simulink model "OpenLoopController"  (R2025b)
settings: configuration reference "VehicleFixed1ms" (kept outside this file)
settings Model: DataDictionary=VirtualMotoTemplate.sldd  ModifiedByFormat=The MathWorks, Inc.  Creator=The MathWorks, Inc.  LastModifiedBy=The MathWorks, Inc.
settings ConfigSetRef: SourceName=VehicleFixed1ms

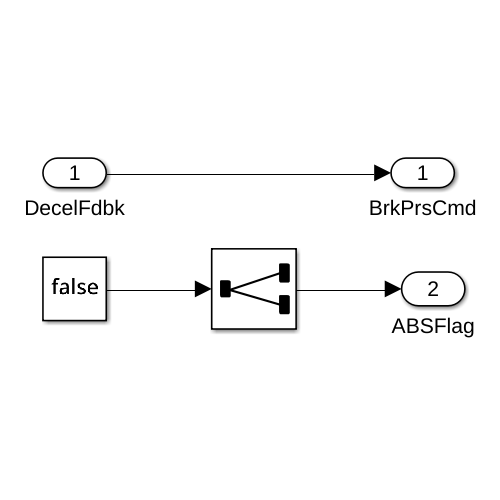
[thumbnail: Simulink's stored preview of the top-level diagram]
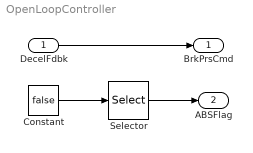
== system OpenLoopController ==
  DecelFdbk : Inport  PortDimensions=2
  Constant : Constant  Value=false
  Selector : Selector  InputPortWidth=1  IndexOptions=Index vector (dialog)  Indices=[1 1]  OutputSizes=1
  BrkPrsCmd : Outport  VectorParamsAs1DForOutWhenUnconnected=off
  ABSFlag : Outport  Port=2
  wires:
  Selector/1 -> ABSFlag/1
  DecelFdbk/1 -> BrkPrsCmd/1
  Constant/1 -> Selector/1
